simulink model "sgMdl_IO424_ResolverMeasurementTest"  (R2024b)
settings: Solver=FixedStepAuto  StartTime=0.0  StopTime=inf  RelTol=1e-3
libraries: dspsrcs4 x3, speedgoatlib_IO424 x2, speedgoatlib_IO107 x1
Description:
  | IO424 - Resolver Measurement
settings Model: ModifiedByFormat=Speedgoat  Creator=Speedgoat  LastModifiedBy=Speedgoat
settings SolverCC: ConcurrentTasks=on  PositivePriorityOrder=on
settings OptimizationCC: BlockReduction=off  OptimizeBlockIOStorage=off
settings DebuggingCC: TasksWithSamePriorityMsg=none
settings HardwareCC: ProdBitPerLong=64  ProdLongLongMode=on  ProdHWDeviceType=Intel->x86-64 (Linux 64)
settings RTWCC: Description=Speedgoat Real-Time Target Machine  SystemTargetFile=speedgoat.tlc  TemplateMakefile=slrealtime_default_tmf  Toolchain=Simulink Real-Time Toolchain  BuildConfiguration=Faster Runs  TargetLang=C++
settings SimulinkRealTimeTargetCC: SubcomponentCodeInterfacePackaging=Reusable function  InstructionSetFMA=off  LogToMDFFile=off  SLRTFileLogMaxRuns=10
settings ConfigComp: CovBoundaryAbsTol=1.0e-5

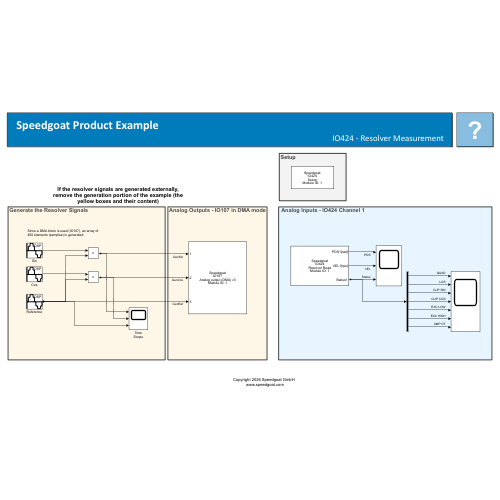
[thumbnail: Simulink's stored preview of the top-level diagram]
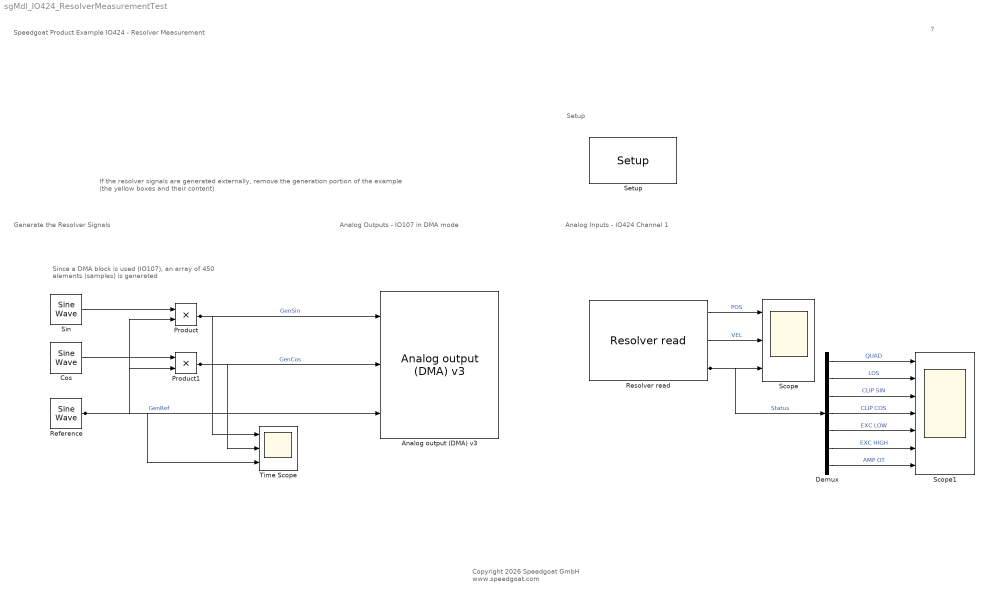
== system sgMdl_IO424_ResolverMeasurementTest ==
  note: Since a DMA block is used (IO107), an array of
      | 450 elements (samples) is generated
  note: If the resolver signals are generated externally, remove the generation portion of the example (the yellow boxes and their content)
  note: Setup
  note: Generate the Resolver Signals
  note: Analog Inputs - IO424 Channel 1
  note: Analog Outputs - IO107 in DMA mode
  note: Speedgoat Product Example
      | IO424 - Resolver Measurement
  note: ?
  note: Copyright 2026 Speedgoat GmbH
      |  www.speedgoat.com
  Analog output (DMA) v3 : speedgoatlib_IO107/Analog output (DMA) v3  id=1  slot=-1  channel_str=[1 10 11]  range=+-10.0  parInit_str=[0]  parReset_str=[1]  autocal=on  gsense=off  clksrc=Internal  syncmode=Async (replay function)  extsync=LVDS  framesize_str=450  samplerate_str=450e3  sampletime_str=-1
      settings: SourceProductName=IO107
  Cos : dspsrcs4/Sine Wave  Amplitude=0.5  Frequency=10  Phase=pi/2  SampleMode=Discrete  OutComplex=Real  CompMethod=Trigonometric fcn  TableSize=Speed  SampleTime=1/450e3  SamplesPerFrame=450  ResetState=Restart at time zero  OutputFrames=off  dataType=double  wordLen=16  udDataType=sfix(16)  fracBitsMode=Best precision  numFracBits=15  OutDataTypeStr=double  LastOutDataTypeStr=double
  Demux : Demux  Outputs=7
  Product : Product
  Product1 : Product
  Reference : dspsrcs4/Sine Wave  Amplitude=4*sqrt(2)  Frequency=1e3  Phase=0  SampleMode=Discrete  OutComplex=Real  CompMethod=Trigonometric fcn  TableSize=Speed  SampleTime=1/450e3  SamplesPerFrame=450  ResetState=Restart at time zero  OutputFrames=off  dataType=double  wordLen=16  udDataType=sfix(16)  fracBitsMode=Best precision  numFracBits=15  OutDataTypeStr=double  LastOutDataTypeStr=double
  Resolver read : speedgoatlib_IO424/Resolver read  parId=1  parShowStatus=on  parShowVelocity=on  parSampleTime=-1  parOutUnits=1  parChannels=1  parCombCh12=0  parCombCh34=0  parNCh=1
      settings: SourceProductName=IO424
  Scope : Scope  NumInputPorts=3
  Scope1 : Scope  NumInputPorts=7
  Setup : speedgoatlib_IO424/Setup  parId=1  parModType=IO424-R (no Synchro)  parPciSlot=-1  parChConf1=Resolver  parChConf2=Disabled  parChConf3=Disabled  parChConf4=Disabled  parPosRdcUnit=Radiants  parCombRdcCh12=off  parCombRdcCh34=on  parChRdcRange1=3.54 Vrms  parChRdcRange2=7.07 Vrms  parChRdcRange3=14.14 Vrms  parChRdcRange4=14.14 Vrms  parPosSynchroUnit=Radiants  parCombSynchroCh34=on  parChSynchroRange3=28 Vrms  parChSynchroRange4=28 Vrms  parCombLvdtCh12=on  parCombLvdtCh34=on  parLvdtRange1A=7.07 Vrms  parLvdtRange1B=14.14 Vrms  parLvdtRange2A=7.07 Vrms  parLvdtRange2B=14.14 Vrms  parLvdtRange3A=7.07 Vrms  parLvdtRange3B=14.14 Vrms  parLvdtRange4A=7.07 Vrms  parLvdtRange4B=14.14 Vrms  parExcEna1=off  parExcVolt1=2  parExcFreq1=1000  parExcEna2=off  parExcVolt2=2  parExcFreq2=1000  parExcEna3=off  parExcVolt3=2  parExcFreq3=1000  parExcEna4=off  parExcVolt4=2  parExcFreq4=1000
      settings: SourceProductName=IO424
  Sin : dspsrcs4/Sine Wave  Amplitude=0.5  Frequency=10  Phase=0  SampleMode=Discrete  OutComplex=Real  CompMethod=Trigonometric fcn  TableSize=Speed  SampleTime=1/450e3  SamplesPerFrame=450  ResetState=Restart at time zero  OutputFrames=off  dataType=double  wordLen=16  udDataType=sfix(16)  fracBitsMode=Best precision  numFracBits=15  OutDataTypeStr=double  LastOutDataTypeStr=double
  Time Scope : Scope  NumInputPorts=3
  wires:
  Resolver read/2 -> Scope/2  "VEL"
  Resolver read/3 -> Demux/1, Scope/3  "Status"
  Resolver read/1 -> Scope/1  "POS"
  Product1/1 -> Analog output (DMA) v3/2, Time Scope/2  "GenCos"
  Product/1 -> Analog output (DMA) v3/1, Time Scope/1  "GenSin"
  Reference/1 -> Analog output (DMA) v3/3, Time Scope/3, Product1/2, Product/2  "GenRef"
  Sin/1 -> Product/1
  Cos/1 -> Product1/1
  Demux/7 -> Scope1/7  "AMP OT"
  Demux/3 -> Scope1/3  "CLIP SIN"
  Demux/4 -> Scope1/4  "CLIP COS"
  Demux/6 -> Scope1/6  "EXC HIGH"
  Demux/1 -> Scope1/1  "QUAD"
  Demux/5 -> Scope1/5  "EXC LOW"
  Demux/2 -> Scope1/2  "LOS"
